simulink model "non_linear"  (R2016a)
settings: Solver=VariableStepAuto  StartTime=0.0  StopTime=600  RelTol=1e-3
libraries: simulink x3
settings Model: Creator=mikae  LastModifiedBy=mikae

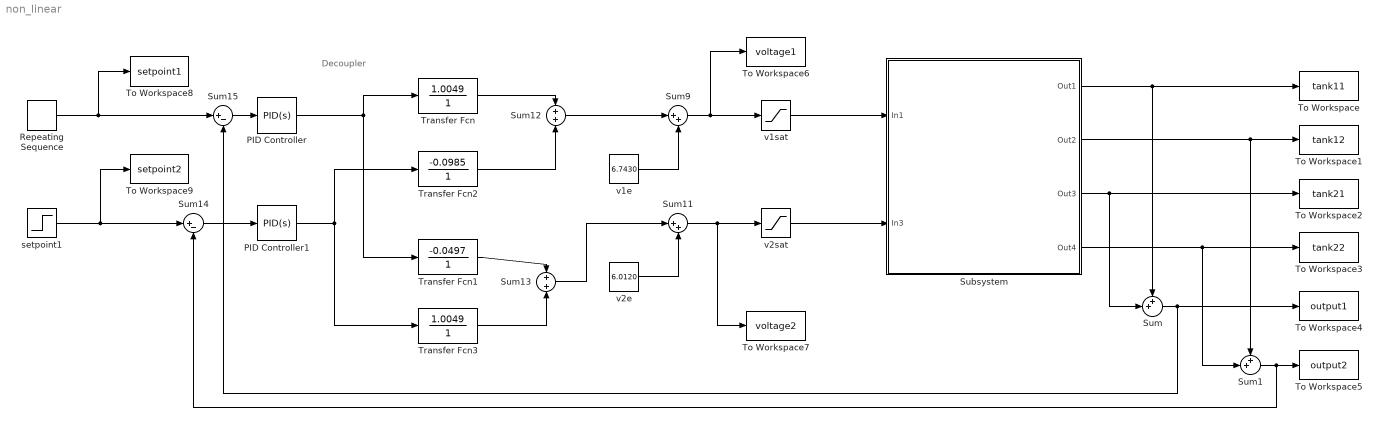
== system non_linear ==
  note: Decoupler
  PID Controller : simulink/Continuous/PID Controller  Controller=PID  TimeDomain=Continuous-time  SampleTime=-1  IntegratorMethod=Forward Euler  FilterMethod=Forward Euler  Form=Ideal  UseFilter=on  ControllerParametersSource=internal  P=10  I=0  D=0  N=100  InitialConditionSource=internal  InitialConditionForIntegrator=0  InitialConditionForFilter=0  ExternalReset=none  LimitOutput=off  UpperSaturationLimit=inf  LowerSaturationLimit=-inf  LinearizeAsGain=on  AntiWindupMode=none  Kb=1  TrackingMode=off  Kt=1  PParamMin=[]  PParamMax=[]  IParamMin=[]  IParamMax=[]  DParamMin=[]  DParamMax=[]  NParamMin=[]  NParamMax=[]  KbParamMin=[]  KbParamMax=[]  KtParamMin=[]  KtParamMax=[]  POutMin=[]  POutMax=[]  IOutMin=[]  IOutMax=[]  DOutMin=[]  DOutMax=[]  NOutMin=[]  NOutMax=[]  KbOutMin=[]  KbOutMax=[]  KtOutMin=[]  KtOutMax=[]  IntegratorOutMin=[]  IntegratorOutMax=[]  FilterOutMin=[]  FilterOutMax=[]  SumOutMin=[]  SumOutMax=[]  SumI1OutMin=[]  SumI1OutMax=[]  SumI2OutMin=[]  SumI2OutMax=[]  SumI3OutMin=[]  SumI3OutMax=[]  SumDOutMin=[]  SumDOutMax=[]  SaturationOutMin=[]  SaturationOutMax=[]  IntegratorContinuousStateAttributes=''  IntegratorStateMustResolveToSignalObject=off  IntegratorRTWStateStorageClass=Auto  FilterContinuousStateAttributes=''  FilterStateMustResolveToSignalObject=off  FilterRTWStateStorageClass=Auto  DifferentiatorICPrevScaledInput=0  DifferentiatorOutMin=[]  DifferentiatorOutMax=[]
  PID Controller1 : simulink/Continuous/PID Controller  Controller=PID  TimeDomain=Continuous-time  SampleTime=-1  IntegratorMethod=Forward Euler  FilterMethod=Forward Euler  Form=Parallel  UseFilter=on  ControllerParametersSource=internal  P=10  I=0  D=0  N=100  InitialConditionSource=internal  InitialConditionForIntegrator=0  InitialConditionForFilter=0  ExternalReset=none  LimitOutput=off  UpperSaturationLimit=inf  LowerSaturationLimit=-inf  LinearizeAsGain=on  AntiWindupMode=none  Kb=1  TrackingMode=off  Kt=1  PParamMin=[]  PParamMax=[]  IParamMin=[]  IParamMax=[]  DParamMin=[]  DParamMax=[]  NParamMin=[]  NParamMax=[]  KbParamMin=[]  KbParamMax=[]  KtParamMin=[]  KtParamMax=[]  POutMin=[]  POutMax=[]  IOutMin=[]  IOutMax=[]  DOutMin=[]  DOutMax=[]  NOutMin=[]  NOutMax=[]  KbOutMin=[]  KbOutMax=[]  KtOutMin=[]  KtOutMax=[]  IntegratorOutMin=[]  IntegratorOutMax=[]  FilterOutMin=[]  FilterOutMax=[]  SumOutMin=[]  SumOutMax=[]  SumI1OutMin=[]  SumI1OutMax=[]  SumI2OutMin=[]  SumI2OutMax=[]  SumI3OutMin=[]  SumI3OutMax=[]  SumDOutMin=[]  SumDOutMax=[]  SaturationOutMin=[]  SaturationOutMax=[]  IntegratorContinuousStateAttributes=''  IntegratorStateMustResolveToSignalObject=off  IntegratorRTWStateStorageClass=Auto  FilterContinuousStateAttributes=''  FilterStateMustResolveToSignalObject=off  FilterRTWStateStorageClass=Auto  DifferentiatorICPrevScaledInput=0  DifferentiatorOutMin=[]  DifferentiatorOutMax=[]
  Repeating Sequence : simulink/Sources/Repeating Sequence  rep_seq_t="[1\t2\t3\t4\t5\t6\t7\t8\t9\t10\t11\t12\t13\t14\t15\t16\t17\t18\t19\t20\t21\t22\t23\t24\t25\t26\t27\t28\t29\t30\t31\t32\t33\t34\t35\t36\t37\t38\t39\t40\t41\t42\t43\t44\t45\t46\t47\t48\t49\t50\t51\t52\t53\t54\t55\t56\t57\t58\t59\t60\t61\t62\t63\t64\t65\t66\t67\t68\t69\t70\t71\t72\t73\t74\t75\t76\t77\t78\t79\t80\t81\t82\t83\t84\t85\t86\t87\t88\t89\t90\t91\t92\t93\t94\t95\t96\t97\t98\t99\t100\t101\t102 ...(+1990 chars)]"  rep_seq_y="[4\t4\t4\t4\t4\t4\t4\t4\t4\t4\t4\t4\t4\t4\t4\t4\t4\t4\t4\t4\t4\t4\t4\t4\t4\t4\t4\t4\t4\t4\t4\t4\t4\t4\t4\t4\t4\t4\t4\t4\t4\t4\t4\t4\t4\t4\t4\t4\t4\t4\t4\t4\t4\t4\t4\t4\t4\t4\t4\t4\t4\t4\t4\t4\t4\t4\t4\t4\t4\t4\t4\t4\t4\t4\t4\t4\t4\t4\t4\t4\t4\t4\t4\t4\t4\t4\t4\t4\t4\t4\t4\t4\t4\t4\t4\t4\t4\t4\t4\t4\t4.21600000000000\t4.43200000000000\t4.64800000000000\t4.86400000000000\t5.08000000000000\t5.29600000000000\t5.51200000000000\t5.72800000000000\t5.94400000000000\t6.16000000000000\t6.37600000000000\t6.59200000000000\t6.80800000000000\t7.02400000000000\t7.24000000000000\t7.45600000000000\t7.67200000000000\t7.88800000000000\t8.10400000000000\t8.32000000000000\t8.53600000000000\t8.75200000000000\t8.96800000000000\t9.18400000000000\t9.40000000000000\t9.61600000000000\t9.83200000000000\t10.0480000000000\t10.2640000000000\t10.4800000000000\t10.6960000000000\t10.9120000000000\t11.1280000000000\t11.3440000000000\t11.5600000000000\t11.7760000000000\t11.9920000000000\t12.2080000000000\t12.4240000000000\t12.6400000000000\t12.8560000000000\t13.0720000000000\t13.2880000000000\t13.5040000000000\t13.7200000000000\t13.9360000000000\t14.1520000000000\t14.3680000000000\t14.5840000000000\t14.8000000000000\t15.0160000000000\t15.2320000000000\t15.4480000000000\t15.6640000000000\t15.8800000000000\t16.0960000000000\t16.3120000000000\t16.5280000000000\t16.7440000000000\t16.9600000000000\t17.1760000000000\t17.3920000000000\t17.6080000000000\t17.8240000000000\t18.0400000000000\t18.2560000000000\t18.4720000000000\t18.6880000000000\t18.9040000000000\t19.1200000000000\t19.3360000000000\t19.5520000000000\t19.7680000000000\t19.9840000000000\t20.2000000000000\t20.4160000000000\t20.6320000000000\t20.8480000000000\t21.0640000000000\t21.2800000000000\t21.4960000000000\t21.7120000000000\t21.9280000000000\t22.1440000000000\t22.3600000000000\t22.5760000000000\t22.7920000000000\t23.0080000000000\t23.2240000000000\t23.4400000000000\t23.6560000000000\t23.8720000000000\t24.0880000000000\t24.3040000000000\t24.5200000000000\t24.7360000000000\t24.9520000000000\t25.1680000000000\t25.3840000000000\t25.6000000000000\t25.8160000000000\t26.0320000000000\t26.2480000000000\t26.4640000000000\t26.6800000000000\t26.8960000000000\t27.1120000000000\t27.3280000000000\t27.5440000000000\t27.7600000000000\t27.9760000000000\t28.1920000000000\t28.4080000000000\t28.6240000000000\t28.8400000000000\t29.0560000000000\t29.2720000000000\t29.4880000000000\t29.7040000000000\t29.9200000000000\t30.1360000000000\t30.3520000000000\t30.5680000000000\t30.7840000000000\t31\t31\t31\t31\t31\t31\t31\t31\t31\t31\t31\t31\t31\t31\t31\t31\t31\t31\t31\t31\t31\t31\t31\t31\t31\t31\t31\t31\t31\t31\t31\t31\t31\t31\t31\t31\t31\t31\t31\t31\t31\t31\t31\t31\t31\t31\t31\t31\t31\t31\t31\t31\t31\t31\t31\t31\t31\t31\t31\t31\t31\t31\t31\t31\t31\t31\t31\t31\t31\t31\t31\t31\t31\t31\t31\t31\t31\t31\t31\t31\t31\t31\t31\t31\t31\t31\t31\t31\t31\t31\t31\t31.2360000000000\t31.4720000000000\t31.7080000000000\t31.9440000000000\t32.1800000000000\t32.4160000000000\t32.6520000000000\t32.8880000000000\t33.1240000000000\t33.3600000000000\t33.5960000000000\t33.8320000000000\t34.0680000000000\t34.3040000000000\t34.5400000000000\t34.7760000000000\t35.0120000000000\t35.2480000000000\t35.4840000000000\t35.7200000000000\t35.9560000000000\t36.1920000000000\t36.4280000000000\t36.6640000000000\t36.9000000000000\t37.1360000000000\t37.3720000000000\t37.6080000000000\t37.8440000000000\t38.0800000000000\t38.3160000000000\t38.5520000000000\t38.7880000000000\t39.0240000000000\t39.2600000000000\t39.4960000000000\t39.7320000000000\t39.9680000000000\t40.2040000000000\t40.4400000000000\t40.6760000000000\t40.9120000000000\t41.1480000000000\t41.3840000000000\t41.6200000000000\t41.8560000000000\t42.0920000000000\t42.3280000000000\t42.5640000000000\t42.8000000000000\t43.0360000000000\t43.2720000000000\t43.5080000000000\t43.7440000000000\t43.9800000000000\t43.7700000000000\t43.5400000000000\t43.3100000000000\t43.0800000000000\t42.8500000000000\t42.6200000000000\t42.3900000000000\t42.1600000000000\t41.9300000000000\t41.7000000000000\t41.4700000000000\t41.2400000000000\t41.0100000000000\t40.7800000000000\t40.5500000000000\t40.3200000000000\t40.0900000000000\t39.8600000000000\t39.6300000000000\t39.4000000000000\t39.1700000000000\t38.9400000000000\t38.7100000000000\t38.4800000000000\t38.2500000000000\t38.0200000000000\t37.7900000000000\t37.5600000000000\t37.3300000000000\t37.1000000000000\t36.8700000000000\t36.6400000000000\t36.4100000000000\t36.1800000000000\t35.9500000000000\t35.7200000000000\t35.4900000000000\t35.2600000000000\t35.0300000000000\t34.8000000000000\t34.5700000000000\t34.3400000000000\t34.1100000000000\t33.8800000000000\t33.6500000000000\t33.4200000000000\t33.1900000000000\t32.9600000000000\t32.7300000000000\t32.5000000000000\t32.2700000000000\t32.0400000000000\t31.8100000000000\t31.5800000000000\t31.3500000000000\t31.1200000000000\t30.8900000000000\t30.6600000000000\t30.4300000000000\t30.2000000000000\t29.9700000000000\t29.7400000000000\t29.5100000000000\t29.2800000000000\t29.0500000000000\t28.8200000000000\t28.5900000000000\t28.3600000000000\t28.1300000000000\t27.9000000000000\t27.6700000000000\t27.4400000000000\t27.2100000000000\t26.9800000000000\t26.7500000000000\t26.5200000000000\t26.2900000000000\t26.0600000000000\t25.8300000000000\t25.6000000000000\t25.3700000000000\t25.1400000000000\t24.9100000000000\t24.6800000000000\t24.4500000000000\t24.2200000000000\t23.9900000000000\t23.7600000000000\t23.5300000000000\t23.3000000000000\t23.0700000000000\t22.8400000000000\t22.6100000000000\t22.3800000000000\t22.1500000000000\t21.9200000000000\t21.6900000000000\t21.4600000000000\t21.2300000000000\t21\t20.7700000000000\t20.5400000000000\t20.3100000000000\t20.0800000000000\t19.8500000000000\t19.6200000000000\t19.3900000000000\t19.1600000000000\t18.9300000000000\t18.7000000000000\t18.4700000000000\t18.2400000000000\t18.0100000000000\t17.7800000000000\t17.5500000000000\t17.3200000000000\t17.0900000000000\t16.8600000000000\t16.6300000000000\t16.4000000000000\t16.1700000000000\t15.9400000000000\t15.7100000000000\t15.4800000000000\t15.2500000000000\t15.0200000000000\t14.7900000000000\t14.5600000000000\t14.3300000000000\t14.1000000000000]"
  Subsystem : Subsystem
  Sum : Sum  Inputs=++|
  Sum1 : Sum  Inputs=++|
  Sum11 : Sum  Inputs=|++
  Sum12 : Sum
  Sum13 : Sum
  Sum14 : Sum  Inputs=|+-
  Sum15 : Sum  Inputs=|+-
  Sum9 : Sum  Inputs=|++
  To Workspace : ToWorkspace  VariableName=tank11  SaveFormat=Timeseries  SampleTime=-1
  To Workspace1 : ToWorkspace  VariableName=tank12  SaveFormat=Timeseries  SampleTime=-1
  To Workspace2 : ToWorkspace  VariableName=tank21  SaveFormat=Timeseries  SampleTime=-1
  To Workspace3 : ToWorkspace  VariableName=tank22  SaveFormat=Timeseries  SampleTime=-1
  To Workspace4 : ToWorkspace  VariableName=output1  SaveFormat=Timeseries  SampleTime=-1
  To Workspace5 : ToWorkspace  VariableName=output2  SaveFormat=Timeseries  SampleTime=-1
  To Workspace6 : ToWorkspace  VariableName=voltage1  SaveFormat=Timeseries  SampleTime=-1
  To Workspace7 : ToWorkspace  VariableName=voltage2  SaveFormat=Timeseries  SampleTime=-1
  To Workspace8 : ToWorkspace  VariableName=setpoint1  SaveFormat=Timeseries  SampleTime=-1
  To Workspace9 : ToWorkspace  VariableName=setpoint2  SaveFormat=Timeseries  SampleTime=-1
  Transfer Fcn : TransferFcn  Numerator=[1.0049]  Denominator=[1]
  Transfer Fcn1 : TransferFcn  Numerator=[-0.0497]  Denominator=[1]
  Transfer Fcn2 : TransferFcn  Numerator=[-0.0985]  Denominator=[1]
  Transfer Fcn3 : TransferFcn  Numerator=[1.0049]  Denominator=[1]
  setpoint1 : Step  Before=22.5  After=26.55  SampleTime=0
  v1e : Constant  Value=6.7430
  v1sat : Saturate  UpperLimit=12  LowerLimit=0
  v2e : Constant  Value=6.0120
  v2sat : Saturate  UpperLimit=12  LowerLimit=0
  wires:
  Sum9/1 -> To Workspace6/1, v1sat/1
  v1e/1 -> Sum9/2
  PID Controller/1 -> Transfer Fcn/1, Transfer Fcn1/1
  PID Controller1/1 -> Transfer Fcn3/1, Transfer Fcn2/1
  Transfer Fcn3/1 -> Sum13/2
  Transfer Fcn1/1 -> Sum13/1
  Transfer Fcn2/1 -> Sum12/2
  Transfer Fcn/1 -> Sum12/1
  Sum12/1 -> Sum9/1
  Sum11/1 -> To Workspace7/1, v2sat/1
  Sum13/1 -> Sum11/1
  v2e/1 -> Sum11/2
  setpoint1/1 -> To Workspace9/1, Sum14/1
  Sum1/1 -> Sum14/2, To Workspace5/1
  Repeating Sequence/1 -> To Workspace8/1, Sum15/1
  Sum/1 -> Sum15/2, To Workspace4/1
  Sum15/1 -> PID Controller/1
  Sum14/1 -> PID Controller1/1
  v1sat/1 -> Subsystem/1(In1)
  v2sat/1 -> Subsystem/2(In3)
  Subsystem/1(Out1) -> Sum/1, To Workspace/1
  Subsystem/2(Out2) -> Sum1/1, To Workspace1/1
  Subsystem/3(Out3) -> Sum/2, To Workspace2/1
  Subsystem/4(Out4) -> Sum1/2, To Workspace3/1

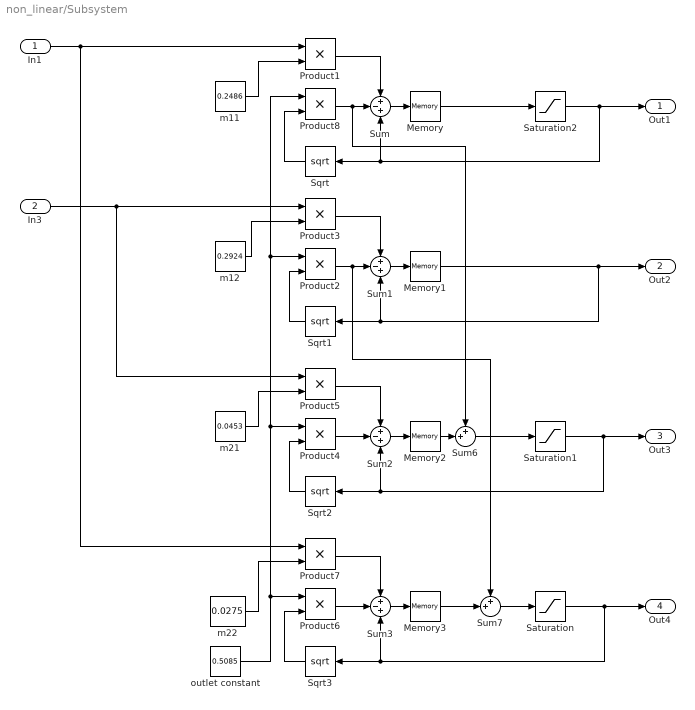
== system non_linear/Subsystem ==
  In1 : Inport
  In3 : Inport  Port=2
  Memory{,1..3} (4 alike) : Memory
  Product{1..8} (8 alike) : Product
  Saturation : Saturate  UpperLimit=30  LowerLimit=0
  Saturation1 : Saturate  UpperLimit=30  LowerLimit=0
  Saturation2 : Saturate  UpperLimit=30  LowerLimit=0
  Sqrt{,1..3} (4 alike) : Sqrt  SaturateOnIntegerOverflow=on
  Sum{,1..3} (4 alike) : Sum  Inputs=+-+
  Sum6 : Sum  Inputs=++|
  Sum7 : Sum  Inputs=++|
  m11 : Constant  Value=0.2486
  m12 : Constant  Value=0.2924
  m21 : Constant  Value=0.0453
  m22 : Constant  Value=0.0275
  outlet constant : Constant  Value=0.5085
  Out1 : Outport
  Out2 : Outport  Port=2
  Out3 : Outport  Port=3
  Out4 : Outport  Port=4
  wires:
  Sum6/1 -> Saturation1/1
  Memory1/1 -> Out2/1, Sum1/3, Sqrt1/1
  Memory/1 -> Saturation2/1
  Sum7/1 -> Saturation/1
  outlet constant/1 -> Product6/1, Product4/1, Product2/1, Product8/1
  m11/1 -> Product1/2
  Product3/1 -> Sum1/1
  Product1/1 -> Sum/1
  m12/1 -> Product3/2
  Product5/1 -> Sum2/1
  Product7/1 -> Sum3/1
  m21/1 -> Product5/2
  m22/1 -> Product7/2
  In1/1 -> Product7/1, Product1/1
  Sum2/1 -> Memory2/1
  Product2/1 -> Sum7/1, Sum1/2
  Memory2/1 -> Sum6/2
  Sum3/1 -> Memory3/1
  In3/1 -> Product5/1, Product3/1
  Sqrt/1 -> Product8/2
  Sqrt2/1 -> Product4/2
  Sum/1 -> Memory/1
  Sqrt3/1 -> Product6/2
  Product8/1 -> Sum6/1, Sum/2
  Sum1/1 -> Memory1/1
  Sqrt1/1 -> Product2/2
  Product4/1 -> Sum2/2
  Product6/1 -> Sum3/2
  Memory3/1 -> Sum7/2
  Saturation/1 -> Out4/1, Sum3/3, Sqrt3/1
  Saturation1/1 -> Out3/1, Sqrt2/1, Sum2/3
  Saturation2/1 -> Out1/1, Sum/3, Sqrt/1
